simulink model "States8_2018a"  (R2018a)
settings: Solver=FixedStepDiscrete  StartTime=0.0  StopTime=0.6  FixedStep=0.1  RelTol=1e-3  EnableMultiTasking=on
settings Model: Creator=bzhan  LastModifiedBy=bzhan
settings SolverCC: AutoInsertRateTranBlk=on
settings DataIOCC: LimitDataPoints=on  ReturnWorkspaceOutputs=on
settings OptimizationCC: LifeSpan=inf
settings DebuggingCC: AllowSymbolicDim=off  SFUnexpectedBacktrackingDiag=warning  SFNoUnconditionalDefaultTransitionDiag=warning  SFExecutionAtInitializationDiag=none
settings CodeAppCC: StateflowObjectComments=on
settings GRTTargetCC: TargetLangStandard=C89/C90 (ANSI)
settings ConfigComp: CovMetricSettings=dw  CovHtmlReporting=on  CovSaveCumulativeToWorkspaceVar=on  CovSaveSingleToWorkspaceVar=on  CovShowResultsExplorer=off  CovExternalEMLEnable=off  CovSFcnEnable=off

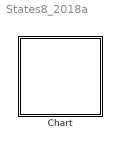
== system States8_2018a ==
  Chart : Stateflow chart  TreatAsAtomicUnit=on

== stateflow chart States8_2018a/Chart ==
  state add
    du: g()
  (default) -> add : {i=1;}
  add -> add : [i<=5]
      | {a(i)=b(i);i=i+1;f("loop")}
  data: s function_input; i local int8; a local =[0,0,0,0,0]; b local =[100,200,300,400,500]
  function f(s):
    | function f(s)
    |   fprintf(s+"\n");
  function g:
    | function g()
    |   fprintf("%.0f,%.0f,%.0f,%.0f,%.0f\n", a(1), a(2), a(3), a(4), a(5));
